simulink model "regcontrol_1ph"  (R2018b)
settings: Solver=VariableStepDiscrete  StartTime=0.0  StopTime=20.0  RelTol=1e-3
values from neighbouring files (symbols this model uses):
  BandWidth = Simulink.Parameter    [start.m]
  BaseVoltage = Simulink.Parameter    [start.m]
  CogenEnabled = false    [regcontrol_emulator.m]    (also in start.m = Simulink.Parameter)
  ElementTerminal = 0    [start.m]
  FPTphase = Simulink.Parameter(FPTphases.DEFAULT)    [regcontrol_emulator.m]    (also in start.m = 1)
  InCogenMode = false    [regcontrol_emulator.m]
  InReverseMode = false    [regcontrol_emulator.m]
  IsReversible = Simulink.Parameter    [start.m]
  LDC_Z = Simulink.Parameter    [start.m]
  MaxTap = 1.10    (= 1.1)    [Transformer.m]
  MinTap = 0.90    (= 0.9)    [Transformer.m]
  PTratio = Simulink.Parameter    [start.m]
  R = 0    [start.m]
  RevBand = Simulink.Parameter    [start.m]
  RevVreg = Simulink.Parameter    [start.m]
  TapLimitPerChange = Simulink.Parameter    [start.m]
  UsingRegulatedBus = Simulink.Parameter    [start.m]
  Vlimit = Simulink.Parameter    [start.m]
  Vreg = Simulink.Parameter    [start.m]
  X = 0    [start.m]
undefined symbols (not defined in the file or in its folder): Armed, ControlledTransformerConnection, ControlledTransformerCurrents, ControlledTransformerPowers, ControlledTransformerVoltages, CTRating, DeltaDirection, Handle, IsInverseTime, LastQueue, LookingForward, m, n, NumConductors, NumPhases, PresentTap, RevBackHandle, RevDelay, ReversePending, RevHandle, revLDC_Z, RevPowerThreshold, revR, revX, TapDelay, TapIncrement, TapWinding, TimeDelay, TimeInSec, VTerminal
(part 1 of 2)
settings Model: Creator=Michael Girbino  LastModifiedBy=Michael Girbino
settings DebuggingCC: LibraryContextMissingDiagnostic=none  SFNoUnconditionalDefaultTransitionDiag=warning  SFOutputUsedAsStateInMooreChartDiag=warning
settings SFSimCC: SimUseLocalCustomCode=off
settings RTWCC: RTWUseLocalCustomCode=off

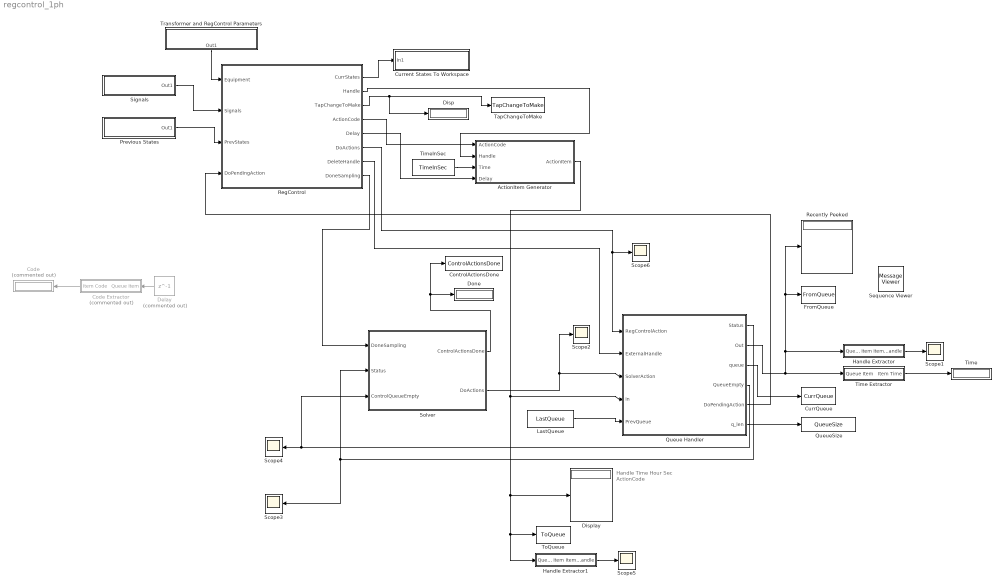
== system regcontrol_1ph ==
  note: Handle
      | Time
      | Hour
      | Sec
      | ActionCode
  ActionItem Generator : Subsystem
  Code : Display  Commented=on
  Code Extractor : Subsystem  Commented=on
  ControlActionsDone : ToWorkspace  VariableName=ControlActionsDone  SaveFormat=Timeseries  SampleTime=-1
  CurrQueue : ToWorkspace  VariableName=CurrQueue  SaveFormat=Structure With Time  SampleTime=1
  Current States To Workspace : Subsystem
  Delay : Delay  Commented=on  DelayLength=1  InitialCondition=0
  Disp : Display
  Display : Display
  Done : Display
  FromQueue : ToWorkspace  VariableName=FromQueue  SaveFormat=Structure With Time  SampleTime=1
  Handle Extractor : Subsystem
  Handle Extractor1 : Subsystem
  LastQueue : Constant  Value=LastQueue  VectorParams1D=off  OutDataTypeStr=double
  Previous States : Subsystem
  Queue Handler : Stateflow chart  TreatAsAtomicUnit=on
  QueueSize : ToWorkspace  VariableName=QueueSize  SaveFormat=Timeseries  SampleTime=-1
      settings: MaxDataPoints=1
  Recently Peeked : Display
  RegControl : Stateflow chart  TreatAsAtomicUnit=on
  Scope{1..6} (6 alike) : Scope
  Sequence Viewer : MessageViewer
  Signals : Subsystem
  Solver : Stateflow chart  TreatAsAtomicUnit=on
  TapChangeToMake : ToWorkspace  VariableName=TapChangeToMake  SaveFormat=Timeseries  SampleTime=-1
      settings: MaxDataPoints=1
  Time : Display
  Time Extractor : Subsystem
  TimeInSec : Constant  Value=TimeInSec  OutDataTypeStr=double
  ToQueue : ToWorkspace  VariableName=ToQueue  SaveFormat=Structure With Time  SampleTime=1
  Transformer and RegControl Parameters : Subsystem
  wires:
  Solver/2(DoActions) -> Scope2/1, Queue Handler/3(SolverAction)
  Queue Handler/1(Status) -> Scope3/1, Solver/2(Status)
  Queue Handler/3(queue) -> CurrQueue/1
  ActionItem Generator/1(ActionItem) -> ToQueue/1, Handle Extractor1/1(Queue Item), Display/1, Queue Handler/4(In)
  Solver/1(ControlActionsDone) -> ControlActionsDone/1, Done/1
  Queue Handler/4(QueueEmpty) -> Solver/3(ControlQueueEmpty), Scope4/1
  TimeInSec/1 -> ActionItem Generator/3(Time)
  LastQueue/1 -> Queue Handler/5(PrevQueue)
  Time Extractor/1(Item Time) -> Time/1
  RegControl/3(TapChangeToMake) -> Disp/1, TapChangeToMake/1
  Queue Handler/2(Out) -> Time Extractor/1(Queue Item), Handle Extractor/1(Queue Item), FromQueue/1, Recently Peeked/1
  Transformer and RegControl Parameters/1(Out1) -> RegControl/1(Equipment)
  RegControl/5(Delay) -> ActionItem Generator/4(Delay)
  Queue Handler/5(DoPendingAction) -> RegControl/4(DoPendingAction)
  RegControl/2(Handle) -> ActionItem Generator/2(Handle)
  RegControl/4(ActionCode) -> ActionItem Generator/1(ActionCode)
  RegControl/8(DoneSampling) -> Solver/1(DoneSampling)
  Signals/1(Out1) -> RegControl/2(Signals)
  Code Extractor/1(Item Code) -> Code/1
  Delay/1 -> Code Extractor/1(Queue Item)
  RegControl/7(DeleteHandle) -> Queue Handler/2(ExternalHandle)
  Previous States/1(Out1) -> RegControl/3(PrevStates)
  RegControl/1(CurrStates) -> Current States To Workspace/1(In1)
  Handle Extractor/1(Item Handle) -> Scope1/1
  Handle Extractor1/1(Item Handle) -> Scope5/1
  RegControl/6(DoActions) -> Scope6/1, Queue Handler/1(RegControlAction)
  Queue Handler/6(q_len) -> QueueSize/1

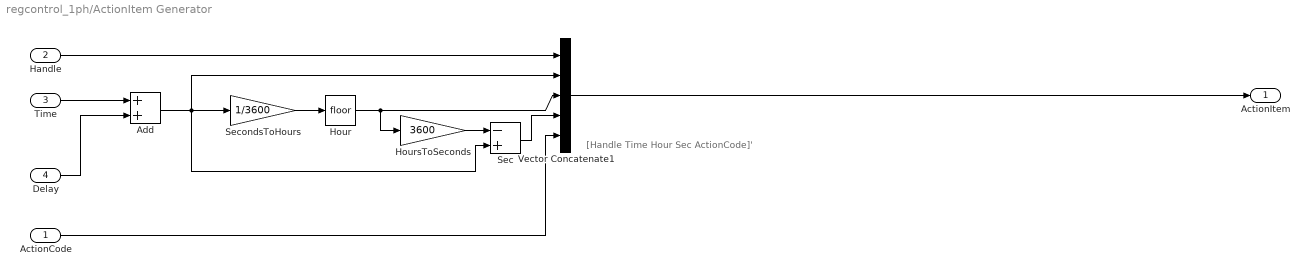
== system regcontrol_1ph/ActionItem Generator ==
  note: [Handle Time Hour Sec ActionCode]'
  ActionCode : Inport
  Handle : Inport  Port=2
  Time : Inport  Port=3
  Delay : Inport  Port=4
  Add : Sum
  Hour : Rounding
  HoursToSeconds : Gain  Gain=3600
  Sec : Sum  Inputs=-+
  SecondsToHours : Gain  Gain=1/3600
  Vector Concatenate1 : Concatenate  NumInputs=5
  ActionItem : Outport
  wires:
  Time/1 -> Add/1
  Hour/1 -> Vector Concatenate1/3, HoursToSeconds/1
  SecondsToHours/1 -> Hour/1
  Vector Concatenate1/1 -> ActionItem/1
  HoursToSeconds/1 -> Sec/1
  Handle/1 -> Vector Concatenate1/1
  Sec/1 -> Vector Concatenate1/4
  ActionCode/1 -> Vector Concatenate1/5
  Delay/1 -> Add/2
  Add/1 -> Sec/2, SecondsToHours/1, Vector Concatenate1/2

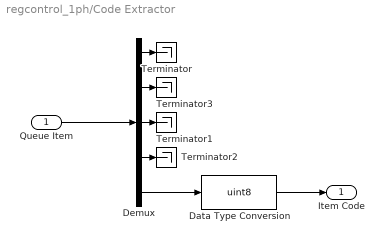
== system regcontrol_1ph/Code Extractor ==
  Queue Item : Inport
  Data Type Conversion : DataTypeConversion  OutDataTypeStr=uint8
  Demux : Demux  Outputs=5
  Terminator{,1..3} (4 alike) : Terminator
  Item Code : Outport
  wires:
  Demux/3 -> Terminator1/1
  Demux/4 -> Terminator2/1
  Demux/1 -> Terminator/1
  Queue Item/1 -> Demux/1
  Demux/5 -> Data Type Conversion/1
  Demux/2 -> Terminator3/1
  Data Type Conversion/1 -> Item Code/1

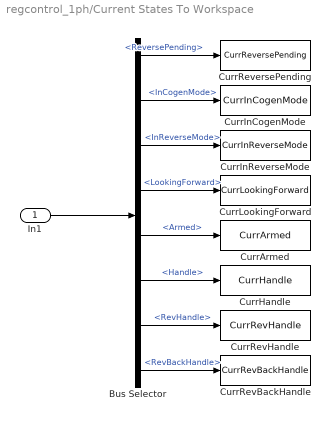
== system regcontrol_1ph/Current States To Workspace ==
  In1 : Inport
  Bus Selector : BusSelector  OutputSignals=ReversePending,InCogenMode,InReverseMode,LookingForward,Armed,Handle,RevHandle,RevBackHandle
  CurrArmed : ToWorkspace  VariableName=CurrArmed  SaveFormat=Timeseries  SampleTime=-1
      settings: MaxDataPoints=1
  CurrHandle : ToWorkspace  VariableName=CurrHandle  SaveFormat=Timeseries  SampleTime=-1
      settings: MaxDataPoints=1
  CurrInCogenMode : ToWorkspace  VariableName=CurrInCogenMode  SaveFormat=Timeseries  SampleTime=-1
      settings: MaxDataPoints=1
  CurrInReverseMode : ToWorkspace  VariableName=CurrInReverseMode  SaveFormat=Timeseries  SampleTime=-1
      settings: MaxDataPoints=1
  CurrLookingForward : ToWorkspace  VariableName=CurrLookingForward  SaveFormat=Timeseries  SampleTime=-1
      settings: MaxDataPoints=1
  CurrRevBackHandle : ToWorkspace  VariableName=CurrRevBackHandle  SaveFormat=Timeseries  SampleTime=-1
      settings: MaxDataPoints=1
  CurrRevHandle : ToWorkspace  VariableName=CurrRevHandle  SaveFormat=Timeseries  SampleTime=-1
      settings: MaxDataPoints=1
  CurrReversePending : ToWorkspace  VariableName=CurrReversePending  SaveFormat=Timeseries  SampleTime=-1
      settings: MaxDataPoints=1
  wires:
  In1/1 -> Bus Selector/1
  Bus Selector/1 -> CurrReversePending/1  "<ReversePending>"
  Bus Selector/2 -> CurrInCogenMode/1  "<InCogenMode>"
  Bus Selector/3 -> CurrInReverseMode/1  "<InReverseMode>"
  Bus Selector/4 -> CurrLookingForward/1  "<LookingForward>"
  Bus Selector/5 -> CurrArmed/1  "<Armed>"
  Bus Selector/6 -> CurrHandle/1  "<Handle>"
  Bus Selector/7 -> CurrRevHandle/1  "<RevHandle>"
  Bus Selector/8 -> CurrRevBackHandle/1  "<RevBackHandle>"

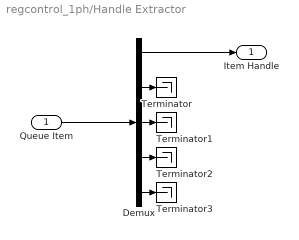
== system regcontrol_1ph/Handle Extractor ==
  Queue Item : Inport
  Demux : Demux  Outputs=5
  Terminator{,1..3} (4 alike) : Terminator
  Item Handle : Outport
  wires:
  Queue Item/1 -> Demux/1
  Demux/4 -> Terminator2/1
  Demux/3 -> Terminator1/1
  Demux/5 -> Terminator3/1
  Demux/1 -> Item Handle/1
  Demux/2 -> Terminator/1

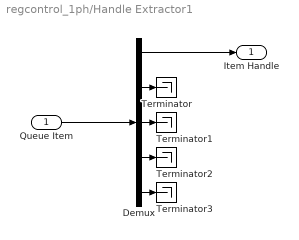
== system regcontrol_1ph/Handle Extractor1 ==
  Queue Item : Inport
  Demux : Demux  Outputs=5
  Terminator{,1..3} (4 alike) : Terminator
  Item Handle : Outport
  wires:
  Demux/2 -> Terminator/1
  Demux/1 -> Item Handle/1
  Demux/5 -> Terminator3/1
  Demux/3 -> Terminator1/1
  Demux/4 -> Terminator2/1
  Queue Item/1 -> Demux/1

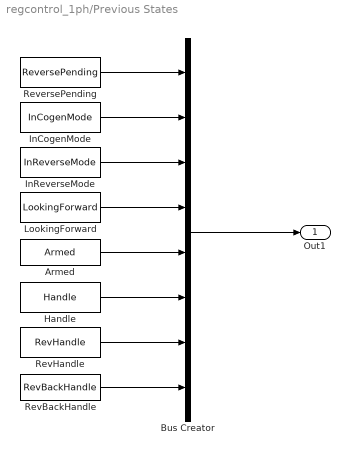
== system regcontrol_1ph/Previous States ==
  Armed : Constant  Value=Armed
  Bus Creator : BusCreator  Inputs=8  OutDataTypeStr=Bus: StatesBus
      settings: InheritFromInputs=off
  Handle : Constant  Value=Handle
  InCogenMode : Constant  Value=InCogenMode
  InReverseMode : Constant  Value=InReverseMode
  LookingForward : Constant  Value=LookingForward
  RevBackHandle : Constant  Value=RevBackHandle
  RevHandle : Constant  Value=RevHandle
  ReversePending : Constant  Value=ReversePending
  Out1 : Outport
  wires:
  Bus Creator/1 -> Out1/1
  ReversePending/1 -> Bus Creator/1
  InCogenMode/1 -> Bus Creator/2
  InReverseMode/1 -> Bus Creator/3
  LookingForward/1 -> Bus Creator/4
  Armed/1 -> Bus Creator/5
  Handle/1 -> Bus Creator/6
  RevHandle/1 -> Bus Creator/7
  RevBackHandle/1 -> Bus Creator/8

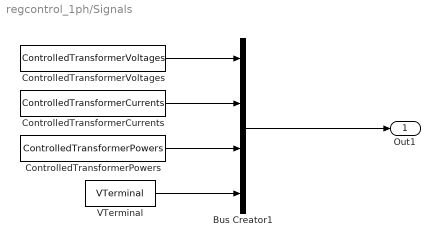
== system regcontrol_1ph/Signals ==
  Bus Creator1 : BusCreator  Inputs=4  OutDataTypeStr=Bus: SignalBus
      settings: InheritFromInputs=off
  ControlledTransformerCurrents : Constant  Value=ControlledTransformerCurrents
  ControlledTransformerPowers : Constant  Value=ControlledTransformerPowers
  ControlledTransformerVoltages : Constant  Value=ControlledTransformerVoltages
  VTerminal : Constant  Value=VTerminal
  Out1 : Outport
  wires:
  Bus Creator1/1 -> Out1/1
  ControlledTransformerPowers/1 -> Bus Creator1/3
  ControlledTransformerVoltages/1 -> Bus Creator1/1
  ControlledTransformerCurrents/1 -> Bus Creator1/2
  VTerminal/1 -> Bus Creator1/4

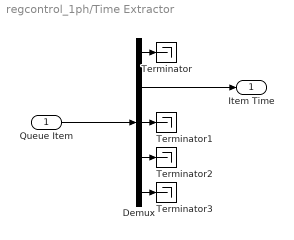
== system regcontrol_1ph/Time Extractor ==
  Queue Item : Inport
  Demux : Demux  Outputs=5
  Terminator{,1..3} (4 alike) : Terminator
  Item Time : Outport
  wires:
  Demux/5 -> Terminator3/1
  Demux/3 -> Terminator1/1
  Demux/4 -> Terminator2/1
  Demux/1 -> Terminator/1
  Demux/2 -> Item Time/1
  Queue Item/1 -> Demux/1

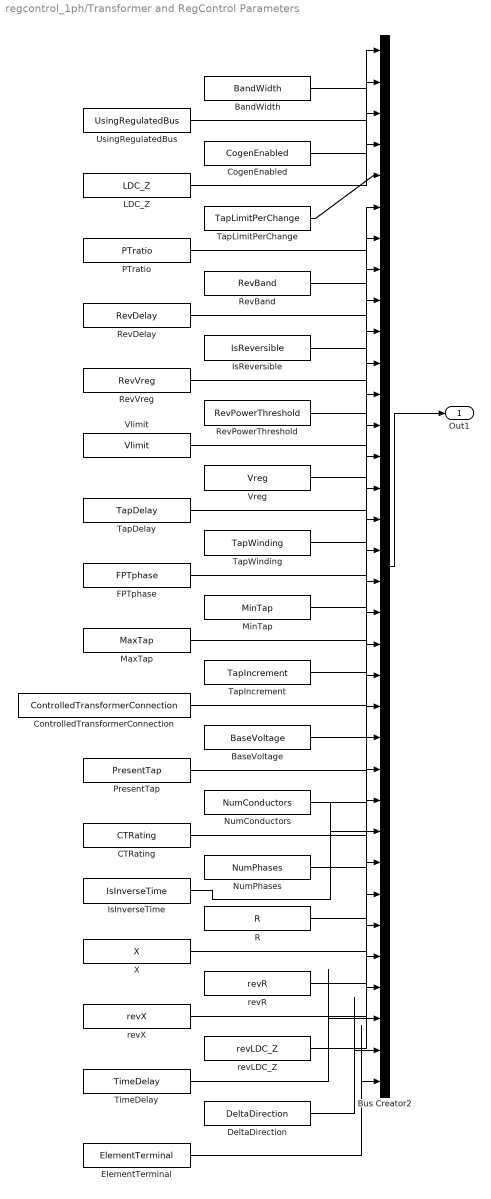
== system regcontrol_1ph/Transformer and RegControl Parameters ==
  BandWidth : Constant  Value=BandWidth
  BaseVoltage : Constant  Value=BaseVoltage
  Bus Creator2 : BusCreator  Inputs=34  OutDataTypeStr=Bus: EquipmentBus
      settings: InheritFromInputs=off
  CTRating : Constant  Value=CTRating
  CogenEnabled : Constant  Value=CogenEnabled
  ControlledTransformerConnection : Constant  Value=ControlledTransformerConnection
  DeltaDirection : Constant  Value=DeltaDirection
  ElementTerminal : Constant  Value=ElementTerminal
  FPTphase : Constant  Value=FPTphase
  IsInverseTime : Constant  Value=IsInverseTime
  IsReversible : Constant  Value=IsReversible
  LDC_Z : Constant  Value=LDC_Z
  MaxTap : Constant  Value=MaxTap
  MinTap : Constant  Value=MinTap
  NumConductors : Constant  Value=NumConductors
  NumPhases : Constant  Value=NumPhases
  PTratio : Constant  Value=PTratio
  PresentTap : Constant  Value=PresentTap
  R : Constant  Value=R
  RevBand : Constant  Value=RevBand
  RevDelay : Constant  Value=RevDelay
  RevPowerThreshold : Constant  Value=RevPowerThreshold
  RevVreg : Constant  Value=RevVreg
  TapDelay : Constant  Value=TapDelay
  TapIncrement : Constant  Value=TapIncrement
  TapLimitPerChange : Constant  Value=TapLimitPerChange
  TapWinding : Constant  Value=TapWinding
  TimeDelay : Constant  Value=TimeDelay
  UsingRegulatedBus : Constant  Value=UsingRegulatedBus
  Vlimit : Constant  Value=Vlimit
  Vreg : Constant  Value=Vreg
  X : Constant  Value=X
  revLDC_Z : Constant  Value=revLDC_Z
  revR : Constant  Value=revR
  revX : Constant  Value=revX
  Out1 : Outport
  wires:
  UsingRegulatedBus/1 -> Bus Creator2/2
  BandWidth/1 -> Bus Creator2/1
  TapWinding/1 -> Bus Creator2/15
  TapDelay/1 -> Bus Creator2/14
  Vreg/1 -> Bus Creator2/13
  Vlimit/1 -> Bus Creator2/12
  RevPowerThreshold/1 -> Bus Creator2/11
  RevVreg/1 -> Bus Creator2/10
  IsReversible/1 -> Bus Creator2/9
  RevDelay/1 -> Bus Creator2/8
  RevBand/1 -> Bus Creator2/7
  PTratio/1 -> Bus Creator2/6
  TapLimitPerChange/1 -> Bus Creator2/5
  LDC_Z/1 -> Bus Creator2/4
  CogenEnabled/1 -> Bus Creator2/3
  Bus Creator2/1 -> Out1/1
  FPTphase/1 -> Bus Creator2/16
  MinTap/1 -> Bus Creator2/17
  MaxTap/1 -> Bus Creator2/18
  TapIncrement/1 -> Bus Creator2/19
  ControlledTransformerConnection/1 -> Bus Creator2/20
  BaseVoltage/1 -> Bus Creator2/21
  PresentTap/1 -> Bus Creator2/22
  NumConductors/1 -> Bus Creator2/23
  CTRating/1 -> Bus Creator2/24
  NumPhases/1 -> Bus Creator2/25
  revLDC_Z/1 -> Bus Creator2/31
  revX/1 -> Bus Creator2/30
  revR/1 -> Bus Creator2/29
  X/1 -> Bus Creator2/28
  R/1 -> Bus Creator2/27
  IsInverseTime/1 -> Bus Creator2/26
  TimeDelay/1 -> Bus Creator2/32
  DeltaDirection/1 -> Bus Creator2/33
  ElementTerminal/1 -> Bus Creator2/34

== stateflow chart regcontrol_1ph/RegControl ==
  settings: enableNonTerminalStates=1
  state MakingTapChange [parallel] [commented out]
    state StaticTapChange [commented out]
      (default) -> (junction 165) [commented out] : {TapChangeToMake = AtLeastOneTap(LocalPendingTapChange, TapIncrement);
          | % reset to no change = change - 1 program will determin if another is needed:
          | LocalPendingTapChange = 0;
          | UpdateArmed(false);}
    state Finished [commented out]
      en: EXIT_TAPCHANGE = true;
    (default) -> (junction 132) [commented out]
    (junction 132) -> (junction 133) [commented out] : % Check to make sure control has not reset:
        | [LocalPendingTapChange == 0]
    (junction 132) -> (junction 163) [commented out]
    (junction 133) -> (junction 135) [commented out] : {UpdateArmed(false);}
    (junction 163) -> StaticTapChange [commented out] : [ControlMode == ControlModes.STATIC]
    (junction 163) -> MakingTapChange.Finished [commented out]
    StaticTapChange -> MakingTapChange.Finished [commented out]
    (junction 135) -> MakingTapChange.Finished [commented out]
  state Sampling [parallel]
    settings: executionOrder=1
    state DetermineReversePendingLookingForward
      state CorrectFalseReversePending
        en:
        if FwdPower < (-1*RevPowerThreshold)
        ReversePending = true;
        DeleteHandle = ...
        Push(ActionCodes.ACTION_REVERSE, ...
        RevDelay);
        RevHandle = DeleteHandle;
        end
      state CorrectTrueReversePending
        en:
        if FwdPower >= (-1*RevPowerThreshold)
        DeleteHandle = RevHandle;
        ReversePending = false;
        DoActions.data = QueueActions.DELETE;
        send(DoActions);
        RevHandle = 0;
        end
      state Finished
        en: GET_VOLTAGE = true;
      (default) -> (junction 599) : {FwdPower = ...
          | -1*real( sum( ControlledTransformerPower((TerminalOffset+1):...
          | (TerminalOffset+NumConductors)) ) );}
          | % Should we reverse?
      (junction 599) -> Sampling.DetermineReversePendingLookingForward.CorrectFalseReversePending [order 1] : [~ReversePending]
      (junction 599) -> (junction 646) [order 2]
      Sampling.DetermineReversePendingLookingForward.CorrectFalseReversePending -> (junction 646)
      (junction 646) -> (junction 594)
      (junction 594) -> Sampling.DetermineReversePendingLookingForward.CorrectTrueReversePending [order 1] : [ReversePending]
      (junction 594) -> (junction 654) [order 2]
      Sampling.DetermineReversePendingLookingForward.CorrectTrueReversePending -> (junction 654)
      (junction 654) -> Sampling.DetermineReversePendingLookingForward.Finished
    state DetermineReversePendingLookingReverseOrCogen
      state CorrectFalseReversePending
        en:
        if FwdPower > RevPowerThreshold
        ReversePending = true;
        % push Reverse Back action to switch back:
        DeleteHandle = ...
        Push(ActionCodes.ACTION_REVERSE, ...
        RevDelay);
        RevBackHandle = DeleteHandle;
        end
      state CorrectTrueReversePending
        en:
        if FwdPower <= RevPowerThreshold
        DeleteHandle = RevBackHandle;
        ReversePending = false;
        % delete Reverse Back action:
        DoActions.data = QueueActions.DELETE;
        send(DoActions);
        RevBackHandle = 0;
        end
      state Finished
        en: REV_NEUTRAL = true;
      (default) -> (junction 620) : {FwdPower = ...
          | -1*real( sum( ControlledTransformerPower((TerminalOffset+1):...
          | (TerminalOffset+NumConductors)) ) );}
          | % If reversed, check if power is back in forward direction
      (junction 620) -> Sampling.DetermineReversePendingLookingReverseOrCogen.CorrectFalseReversePending [order 1] : [~ReversePending]
      (junction 620) -> (junction 621) [order 2]
      Sampling.DetermineReversePendingLookingReverseOrCogen.CorrectFalseReversePending -> (junction 621)
      (junction 621) -> (junction 624)
      (junction 624) -> Sampling.DetermineReversePendingLookingReverseOrCogen.CorrectTrueReversePending [order 1] : [ReversePending]
      (junction 624) -> (junction 650) [order 2]
      Sampling.DetermineReversePendingLookingReverseOrCogen.CorrectTrueReversePending -> (junction 650)
      (junction 650) -> Sampling.DetermineReversePendingLookingReverseOrCogen.Finished
    state ReverseNeutralCase
      state Finished
        en:
        GET_VOLTAGE = true;
      state ReverseNeutralTapChange
        en:
        PendingTapChange = ...
        round( (1.0 - double(TapWinding)) / TapIncrement ) * TapIncrement;
        if PendingTapChange ~= 0.0 && ~Armed
        Push(ActionCodes.ACTION_TAPCHANGE, TapDelay);
        Armed = true;
        end
      state Exiting
        en: EXIT = true;
      (default) -> (junction 592)
      (junction 592) -> (junction 637) [order 1] : % tap change not specified as needed:
          | [~Armed]
      (junction 592) -> Sampling.ReverseNeutralCase.Finished [order 2]
      (junction 637) -> (junction 614) : {PendingTapChange = 0.0;}
      (junction 614) -> (junction 638) [order 1] : [abs(PresentTap - 1.0) < EPSILON]
      (junction 614) -> Exiting [order 2]
      (junction 638) -> ReverseNeutralTapChange
      ReverseNeutralTapChange -> (junction 649)
      (junction 649) -> Exiting
    state GetVoltage
      en:
      if UsingRegulatedBus
      GetRegulatedBusVoltage; % stores voltages in VBuffer
      else
      VBuffer = ControlledTransformerWindingVoltages((TerminalOffset+1):(TerminalOffset+NumPhases));
      end
      Vcontrol = GetControlVoltage; % operates on VBuffer
    state DetermineVlocalbus
      state Finished
        en: GET_VOLTAGEWLDC = true;
      (default) -> (junction 689)
      (junction 689) -> (junction 691) [order 1] : % Voltage limit for bus connected to regulated winding; default = 0.0 (inactive)
          | [VlimitActive]
      (junction 689) -> Sampling.DetermineVlocalbus.Finished [order 2] : {Vlocalbus = 0.0;}
      (junction 691) -> (junction 683)
      (junction 683) -> (junction 692) [order 1] : % when controlled transformer is different from LDC PTransformer
          | [UsingRegulatedBus]
      (junction 683) -> (junction 696) [order 2] : % controlled transformer is
          | % the LDC PTransformer
          | {Vlocalbus = abs(Vcontrol);}
      (junction 692) -> (junction 714) : {%ControlledTransformer.GetWindingVoltages(ElementTerminal, VBuffer);
          | Vlocalbus = abs( VBuffer(1) / PTRatio );}
      (junction 714) -> (junction 696)
      (junction 696) -> (junction 675)
      (junction 675) -> Sampling.DetermineVlocalbus.Finished
    state GetVoltageWithLDC
      state RX_LDCmode
        en:
        if InReverseMode || InCogenMode
        VLDC = complex(revR, revX) * ...
        complex( real(ILDC), imag(ILDC) );
        else
        VLDC = complex(R, X) * ...
        complex( real(ILDC), imag(ILDC) );
        end
      state Z_LDCmode
        en:
        if InReverseMode || InCogenMode
        Vcontrol = abs(Vcontrol) - abs(ILDC) * revLDC_Z;
        else
        Vcontrol = abs(Vcontrol) - abs(ILDC) * LDC_Z;
        end
      state Finished
        en: GET_TEST_VALUES = true;
      (default) -> (junction 771) : {% Convert current to control current by CTRating:
          | ILDC = ControlledTransformerCurrents(TerminalOffset + ControlledPhase) / CTRating;}
      (junction 771) -> RX_LDCmode [order 1] : % Standard R, X LDC
          | [LDC_Z == 0.0]
      (junction 771) -> Z_LDCmode [order 2] : % Beckwith LDC_Z control mode
      RX_LDCmode -> (junction 872)
      Z_LDCmode -> Sampling.GetVoltageWithLDC.Finished
      (junction 872) -> Sampling.GetVoltageWithLDC.Finished
    state GetTestValues
      en:
      Vactual = abs(Vcontrol);
      if InReverseMode
      Vactual = Vactual / PresentTap;
      VregTest = RevVreg;
      BandTest = RevBandwidth;
      else
      VregTest = Vreg;
      BandTest = Bandwidth;
      end
    state DetermineTapChangeIsNeeded
      en:
      if abs(VregTest - Vactual) > BandTest/2.0
      TapChangeIsNeeded = true;
      else
      TapChangeIsNeeded = false;
      end
    state MakeTapChange
      state GetVboostFromVlimit
        en:
        if Vlocalbus > Vlimit
        Vboost = Vlimit - Vlocalbus;
        end
      state TapChangeUp
        en:
        if PresentTap < MaxTap
        Push(ActionCodes.ACTION_TAPCHANGE, ...
        ComputeTimeDelay(Vactual));
        Armed = true;
        end
      state TapChangeDown
        en:
        if PresentTap > MinTap
        Push(ActionCodes.ACTION_TAPCHANGE, ...
        ComputeTimeDelay(Vactual));
        Armed = true;
        end
      state Finished
        en: FINISHED = true;
      (default) -> (junction 720) : % compute tapchange:
          | {Vboost = VregTest - Vactual;}
      (junction 720) -> (junction 766) [order 1] : [VlimitActive]
      (junction 720) -> (junction 723) [order 2]
      (junction 766) -> GetVboostFromVlimit
      GetVboostFromVlimit -> (junction 724)
      (junction 724) -> (junction 723)
      (junction 723) -> (junction 728) : {% PU winding boost needed:
          | BoostNeeded = Vboost * PTRatio / BaseVoltage;
          | Increment = TapIncrement;
          | % quantize to an increment:
          | PendingTapChange = ...
          | round(BoostNeeded/Increment)*Increment;
          | }
      (junction 728) -> (junction 731) : % send initial tap change message to ControlQueue, add delay time to solution control queue:
      (junction 731) -> (junction 817) [order 1] : % only changes 1 tap at a time:
          | [PendingTapChange ~= 0.0 && ~Armed]
      (junction 731) -> Sampling.MakeTapChange.Finished [order 2]
      (junction 817) -> (junction 810) : % see of any tap change is possible in desired direction (not saturated):
      (junction 810) -> TapChangeUp [order 1] : % going up:
          | [PendingTapChange > 0.0]
      (junction 810) -> TapChangeDown [order 2]
      TapChangeUp -> (junction 819)
      TapChangeDown -> (junction 820)
      (junction 820) -> Sampling.MakeTapChange.Finished
      (junction 819) -> (junction 820)
    state Finished
      en:
      WriteStatesToOutput;
      send(DoneSampling);
    (default) -> (junction 822) : {AssignEquipmentToLocals;
        | AssignSignalsToLocals;
        | AssignStatesToLocals;}
    (junction 822) -> (junction 815) [order 1] : [TapLimitPerChange ~= 0]
    (junction 815) -> (junction 826)
    (junction 822) -> (junction 807) [order 2]
    (junction 826) -> (junction 823) [order 1] : [~UsingRegulatedBus]
    (junction 826) -> (junction 818) [order 2]
    (junction 823) -> (junction 787)
    (junction 787) -> (junction 832) [order 1] : [IsReversible || CogenEnabled]
    (junction 787) -> (junction 792) [order 2]
    (junction 832) -> (junction 828)
    (junction 828) -> DetermineReversePendingLookingForward [order 1] : [LookingForward && ~InCogenMode]
    (junction 828) -> DetermineReversePendingLookingReverseOrCogen [order 2]
    DetermineReversePendingLookingForward -> (junction 825) : [GET_VOLTAGE]
    DetermineReversePendingLookingReverseOrCogen -> (junction 844) : [REV_NEUTRAL]
    (junction 844) -> ReverseNeutralCase [order 1] : % mode for which tap change may be executed,
        | % but no reversal made:
        | [ReverseNeutral]
    (junction 844) -> (junction 806) [order 2]
    ReverseNeutralCase -> (junction 806) [order 2] : [GET_VOLTAGE]
    (junction 806) -> (junction 808)
    ReverseNeutralCase -> (junction 829) [order 1] : [EXIT]
    (junction 792) -> (junction 818)
    (junction 808) -> (junction 792)
    (junction 825) -> (junction 808)
    (junction 818) -> GetVoltage
    (junction 829) -> (junction 807)
    (junction 807) -> (junction 816)
    GetVoltage -> DetermineVlocalbus
    DetermineVlocalbus -> (junction 845) : [GET_VOLTAGEWLDC]
    (junction 845) -> GetVoltageWithLDC [order 1] : % line drop compensation, but not using regulated bus
        | [~UsingRegulatedBus && LDCActive]
    (junction 845) -> (junction 809) [order 2]
    GetVoltageWithLDC -> (junction 839) : [GET_TEST_VALUES]
    (junction 839) -> (junction 809)
    (junction 809) -> GetTestValues
    GetTestValues -> DetermineTapChangeIsNeeded
    DetermineTapChangeIsNeeded -> (junction 788)
    (junction 788) -> MakeTapChange [order 1] : [TapChangeIsNeeded]
    (junction 788) -> (junction 813) [order 2]
    MakeTapChange -> (junction 837) : [FINISHED]
    (junction 837) -> (junction 813)
    (junction 813) -> Sampling.Finished
    (junction 816) -> Sampling.Finished : {PendingTapChange = 0;}
  state Execution [parallel]
    settings: executionOrder=2
    state Asleep
    state ParseAction
      en: Code = DoPendingAction.data;
      discard(DoPendingAction);
      length(DoPendingAction);
    state MakingTapChange
      en:
      if PendingTapChange ~= 0
      TapChangeToMake = AtLeastOneTap(PendingTapChange);
      PendingTapChange = 0;
      Armed = false;
      end
    state Reversing
      state FlipCogen
        en:
        if InCogenMode
        InCogenMode = false;
        else
        InCogenMode = true;
        end
      state FlipReverse
        en:
        if InReverseMode
        InReverseMode = false;
        else
        InReverseMode = true;
        end
      state Finished
        en:
        ReversePending = false;
        EXIT_REVERSE = true;
      (default) -> (junction 229)
      (junction 229) -> (junction 230) [order 1] : [ReversePending]
      (junction 229) -> Execution.Reversing.Finished [order 2]
      (junction 230) -> (junction 242)
      (junction 242) -> (junction 238) [order 1] : [CogenEnabled]
      (junction 242) -> FlipReverse [order 2]
      (junction 238) -> FlipCogen : % Cogen mode takes precedence if present
      FlipReverse -> (junction 240)
      FlipCogen -> (junction 245)
      (junction 240) -> Execution.Reversing.Finished
      (junction 245) -> (junction 240)
    state Finished
      en: WriteStatesToOutput;
    (default) -> Asleep
    Asleep -> ParseAction : DoPendingAction
    ParseAction -> (junction 115)
    (junction 115) -> Execution.MakingTapChange [order 1] : [Code == ActionCodes.ACTION_TAPCHANGE]
    (junction 115) -> (junction 119) [order 2]
    Execution.MakingTapChange -> (junction 122)
    (junction 119) -> Reversing [order 1] : [Code == ActionCodes.ACTION_REVERSE]
    (junction 119) -> (junction 123) [order 2]
    Reversing -> (junction 122) : [EXIT_REVERSE]
    (junction 122) -> (junction 124)
    (junction 124) -> (junction 123)
    (junction 123) -> Execution.Finished
  state ChangeToMake = AtLeastOneTap(ProposedChange) [function]
    note: Called in STATIC mode
        | Changes 70% of the way but at least one tap, subject to maximum allowable tap change
    (default) -> (junction 283) : {NumTaps = floor(0.7 * abs(ProposedChange)/TapIncrement);}
    (junction 283) -> (junction 284) [order 1] : [NumTaps == 0]
    (junction 283) -> (junction 285) [order 2]
    (junction 284) -> (junction 286) : {NumTaps = 1.0;} % At least 1 tap
    (junction 286) -> (junction 285)
    (junction 285) -> (junction 293)
    (junction 293) -> (junction 290) [order 1] : [NumTaps > TapLimitPerChange]
    (junction 293) -> (junction 294) [order 2]
    (junction 290) -> (junction 295) : {NumTaps = double(TapLimitPerChange);} % Bound by maximum
    (junction 295) -> (junction 294)
    (junction 294) -> (junction 302) : {LastChange = NumTaps;}
    (junction 302) -> (junction 303) [order 1] : % Check sign on change:
        | [ProposedChange > 0]
    (junction 302) -> (junction 304) [order 2] : {ChangeToMake = ...
        | -1*double(NumTaps)*TapIncrement;
        | LastChange = -1*NumTaps;}
    (junction 303) -> (junction 305) : {ChangeToMake =...
        |  double(NumTaps)*TapIncrement;}
    (junction 305) -> (junction 304)
    (junction 304) -> (junction 306)
  state Result = GetControlVoltage [function]
    note: GetControlVoltage
        | Called when voltage is sampled from the same transformer whose taps are controlled.
        | Returns the voltage which will be used to decide tap changes. Also changes the ControlledPhase if it is different from FPTphase.
    note: FPTphase is max phase.
        |
        | VControl is taken from the phase with the greatest voltage.
        |
        | ControlledPhase becomes that phase.
    note: FPTphase is min phase.
        |
        | VControl is taken from the phase with the least voltage.
        |
        | ControlledPhase becomes that phase.
    (default) -> (junction 496)
    (junction 496) -> (junction 486) [order 1] : [FPTphase == uint8(FPTphases.MAXPHASE)]
        | % controlled phase is that with greatest |V|
    (junction 496) -> (junction 517) [order 2]
    (junction 486) -> (junction 523) : {ControlledPhase = 1;
        | % abs is equivalent to Cabs:
        | V = abs( VBuffer(ControlledPhase) );}
        | % Iteration through remaining phases:
    (junction 510) -> (junction 489) [order 1] : [ii <= NumPhases]
    (junction 489) -> (junction 485)
    (junction 523) -> (junction 510) : {ii = uint8(2);}
    (junction 485) -> (junction 515) [order 1] : [abs( VBuffer(ControlledPhase)) > V]
        | % if it's GREATER, make it the new V
    (junction 485) -> (junction 522) [order 2]
    (junction 515) -> (junction 516) : {V = abs( VBuffer(ii) );
        | ControlledPhase = ii;}
    (junction 487) -> (junction 510) : {ii = ii+1;}
    (junction 510) -> (junction 534) [order 2] : {Result = VBuffer(ControlledPhase) / PTRatio;
        | % Complex divided by real
        | }
    (junction 516) -> (junction 522)
    (junction 522) -> (junction 487)
    (junction 534) -> (junction 527)
    (junction 527) -> (junction 519)
    (junction 517) -> (junction 533) [order 1] : [FPTphase == uint8(FPTphases.MINPHASE)]
        | % controlled phase is that with least |V|
    (junction 533) -> (junction 535) : {ControlledPhase = 1;
        | % abs is equivalent to Cabs:
        | V = abs( VBuffer(ControlledPhase) );}
        | % Iteration through remaining phases:
    (junction 517) -> (junction 1027) [order 2] : % Default case: use specified phase,
        | % as long as it's feasible
    (junction 513) -> (junction 537) [order 1] : [ii <= NumPhases]
    (junction 537) -> (junction 488)
    (junction 535) -> (junction 513) : {ii = uint8(2);}
    (junction 1027) -> (junction 1028) [order 1] : [FPTphase > NumPhases]
    (junction 488) -> (junction 504) [order 1] : [abs( VBuffer(ControlledPhase)) < V]
        | % if it's LESS, make it the new V
    (junction 1027) -> (junction 1029) [order 2] : {FPTphase = max(FPTphase, 1);}
    (junction 1028) -> (junction 1030) : {FPTphase = 1;}
    (junction 488) -> (junction 514) [order 2]
    (junction 504) -> (junction 507) : {V = abs( VBuffer(ii) );
        | ControlledPhase = ii;}
    (junction 518) -> (junction 513) : {ii = ii+1;}
    (junction 513) -> (junction 536) [order 2] : {Result = VBuffer(ControlledPhase) / PTRatio;
        | % Complex divided by real
        | }
    (junction 507) -> (junction 514)
    (junction 514) -> (junction 518)
    (junction 1030) -> (junction 1029)
    (junction 1029) -> (junction 497) : {Result = VBuffer(FPTphase) / PTRatio;
        | ControlledPhase = FPTphase;}
    (junction 536) -> (junction 519)
    (junction 519) -> (junction 502)
    (junction 502) -> (junction 497)
    (junction 497) -> (junction 498)
  state Result = ComputeTimeDelay(Vavg) [function]
    (default) -> (junction 477)
    (junction 477) -> (junction 481) [order 1] : [IsInverseTime]
    (junction 477) -> (junction 482) [order 2] : % determines which regulator control will act first,
        | % default is 15s
        | {Result = TimeDelay;}
    (junction 481) -> (junction 483) : % TimeDelay is adjusted inversely proportional to
        | % the amount that voltage is outside the band,
        | % down to 10 percent of specified time delay
        | % (Further out of band = band - 1> less time delay)
        | {Result = TimeDelay / min(10.0, 2.0*abs(Vreg - Vavg)/Bandwidth);}
    (junction 483) -> (junction 482)
    (junction 482) -> (junction 474)
  state AssignEquipmentToLocals [function]
    (default) -> (junction 550) : {
        | BandWidth = Equipment.BandWidth;
        | UsingRegulatedBus = Equipment.UsingRegulatedBus;
        | CogenEnabled = Equipment.CogenEnabled;
        | LDC_Z = Equipment.LDC_Z;
        | TapLimitPerChange = Equipment.TapLimitPerChange;
        | PTRatio = Equipment.PTratio;
        | RevBand = Equipment.RevBand;
        | RevDelay = Equipment.RevDelay;
        | IsReversible = Equipment.IsReversible;
        | RevVreg = Equipment.RevVreg;
        | RevPowerThreshold = Equipment.RevPowerThreshold;
        | Vlimit = Equipment.Vlimit;
        | Vreg = Equipment.Vreg;
        | TapDelay = Equipment.TapDelay;
        | TapWinding = Equipment.TapWinding;
        | FPTphase = Equipment.FPTphase;
        |
        | MinTap = Equipment.MinTap;
        | MaxTap = Equipment.MaxTap;
        | TapIncrement = Equipment.TapIncrement;
        | ControlledTransformerConnection = Equipment.ControlledTransformerConnection;
        | BaseVoltage = Equipment.BaseVoltage;
        | NumConductors = Equipment.NumConductors;
        | NumPhases = Equipment.NumPhases;
        | CTRating = Equipment.CTRating;
        | IsInverseTime = Equipment.IsInverseTime;
        |
        | R = Equipment.R;
        | X = Equipment.X;
        | revR = Equipment.revR;
        | revX = Equipment.revX;
        | revLDC_Z = Equipment.revLDC_Z;
        | TimeDelay = Equipment.TimeDelay;
        |
        | % From Script:
        | TapWinding = Equipment.TapWinding;
        | TapIncrement = Equipment.TapIncrement;
        | TapDelay = Equipment.TapDelay;
        | CogenEnabled = Equipment.CogenEnabled;
        | PresentTap = Equipment.PresentTap;
        | TapLimitPerChange = Equipment.TapLimitPerChange;
        | ElementTerminal = Equipment.ElementTerminal;
        | DeltaDirection = Equipment.DeltaDirection;
        | }
    (junction 550) -> (junction 548) [order 1] : [R~=0 || X~=0 || LDC_Z ~=0]
    (junction 550) -> (junction 555) [order 2] : {LDCActive = false;}
    (junction 548) -> (junction 552) : {LDCActive = true;}
    (junction 552) -> (junction 555)
    (junction 555) -> (junction 547)
  state h = Push(CodeVal, DelayVal) [function]
    (default) -> (junction 462) : {ActionCode = double(CodeVal);
        | Delay = DelayVal;
        | DoActions.data = QueueActions.PUSH;
        | send(DoActions);
        | h = uint8(Handle);
        | Handle = Handle + double(1);
        | }
  state AssignSignalsToLocals [function]
    (default) -> (junction 940) : {ControlledTransformerWindingVoltages = Signals.ControlledTransformerVoltages;
        | ControlledTransformerPower = Signals.ControlledTransformerPowers;
        | ControlledTransformerCurrents = Signals.ControlledTransformerCurrents;
        | VTerminal = Signals.VTerminal;
        |
        | TerminalOffset = NumConductors*(ElementTerminal - 1);
        | VBuffer = zeros(NumPhases, 1);}
  state AssignStatesToLocals [function]
    (default) -> (junction 943) : {ReversePending = PrevStates.ReversePending;
        | InCogenMode = PrevStates.InCogenMode;
        | InReverseMode = PrevStates.InReverseMode;
        | LookingForward = PrevStates.LookingForward;
        | Armed = PrevStates.Armed;
        | Handle = double(PrevStates.Handle);
        | RevHandle = PrevStates.RevHandle;
        | RevBackHandle = PrevStates.RevBackHandle;
        | }
  state GetRegulatedBusVoltage [function]
    (junction 989) -> (junction 998) [order 1] : [ii <= NumPhases]
    (default) -> (junction 989) : {ii = uint8(1);}
    (junction 998) -> (junction 1002)
    (junction 1002) -> (junction 991) [order 1] : [ControlledTransformerConnection == Connections.DELTA]
    (junction 1002) -> (junction 1015) [order 2]
    (junction 991) -> (junction 992) : {rotIdx = RotatePhases(ii, NumPhases, DeltaDirection);
        | VBuffer(ii) = VTerminal(TerminalOffset+ii) - ...
        | VTerminal(TerminalOffset+rotIdx);}
    (junction 1015) -> (junction 1007) [order 1] : [ControlledTransformerConnection == ...
        | Connections.WYE]
    (junction 1015) -> (junction 1017) [order 2]
    (junction 1007) -> (junction 990) : {VBuffer(ii) = VTerminal(TerminalOffset+ii);}
    (junction 997) -> (junction 989) : {ii = ii+1;}
    (junction 989) -> (junction 1005) [order 2]
    (junction 990) -> (junction 1017)
    (junction 992) -> (junction 990)
    (junction 1017) -> (junction 997)
  state WriteStatesToOutput [function]
    (default) -> (junction 947) : {CurrStates.ReversePending = ReversePending;
        | CurrStates.InCogenMode = InCogenMode;
        | CurrStates.InReverseMode = InReverseMode;
        | CurrStates.LookingForward = LookingForward;
        | CurrStates.Armed = Armed;
        | CurrStates.Handle = uint8(Handle);
        | CurrStates.RevHandle = RevHandle;
        | CurrStates.RevBackHandle = RevBackHandle;
        | }
  data: ProposedChange function_input; ChangeToMake function_output; NumTaps local double; Result function_output; Vavg function_input; Result function_output; CodeVal function_input; DelayVal function_input; h function_output; idx function_input; newIdx function_output; NPhases function_input; DeltaDir function_input; CurrStates output Bus: StatesBus; Equipment input Bus: EquipmentBus; Signals input Bus: SignalBus; PrevStates input Bus: StatesBus; Handle output double =0; EXIT_REVERSE local boolean =false; InReverseMode local boolean =false; ReversePending local boolean; InCogenMode local boolean =false; DoPendingAction input double; TapWinding local uint8; TapIncrement local double; TapDelay local double; CogenEnabled local boolean =false; TapChangeToMake output double; PendingTapChange local double =double(0); TapLimitPerChange local uint8 =uint8(16); ActionCode output double; Delay output double =0; DoActions output Enum: QueueActions; DeleteHandle output uint8 size=[1] =uint8(0); DoneSampling output boolean =true; Armed local boolean =false; PresentTap local double; Vactual local double =0; Vcontrol local double =complex(0); FPTphase local uint8 size=[1]; VBuffer local double size=[3 1]; NumPhases local uint8 size=[1]; ControlledPhase local uint8 size=[1] =uint8(1); PTRatio local double =60; IsInverseTime local boolean; TimeDelay local double; Vreg local double =120; Bandwidth local double =3; revR local double =0; RevVreg local double =120; revX local double =0; ControlledTransformerConnection local uint8 size=[1]; ControlledTransformerCurrents local double; ControlledTransformerPower local double; ControlledTransformerWindingVoltages local double size=[4 1]; CTRating local double; MaxTap local double; MinTap local double; Vlimit local double =0; RevDelay local double; revLDC_Z local double =0; RevPowerThreshold local double; RevBandwidth local double =3; ElementTerminal local uint8 size=[1] =uint8(1); LDCActive local boolean =false; VlimitActive local boolean =false; Increment local double =0; IsReversible local boolean =false; LookingForward local boolean =false; ReverseNeutral local boolean =false; NumConductors local uint8 size=[1]; BaseVoltage local double; UsingRegulatedBus local boolean =false; VLDC local double =complex(0); FINISHED local boolean =false; VregTest local double =0; BandTest local double =0; EXIT local boolean =false; ILDC local double =complex(0); Vboost local double =0; FwdPower local double =0; GET_TEST_VALUES local boolean =false; GET_VOLTAGE local boolean =false; GET_VOLTAGEWLDC local boolean =false; Vlocalbus local double =0; BoostNeeded local double =0; RevBackHandle local uint8 size=[1] =uint8(0); REV_NEUTRAL local boolean =false; TapChangeIsNeeded local boolean =false; LDC_Z local double =0; R local double =0; X local double =0; EPSILON local double =1.0e-12; RevHandle local uint8 size=[1] =uint8(0); LastChange local double; DeltaDirection local uint8; VTerminal local double size=[4 1]; TerminalOffset local uint8 =uint8(0); Code local double size=[1 1]
  function newIdx = RotatePhases(idx, NPhases, DeltaDir):
    | function newIdx = RotatePhases(idx, NPhases, DeltaDir)
    |     dd = int8(1);
    |     
    |     switch(DeltaDir)
    |         case DeltaDirs.FORWARD
    |             dd = int8(1);
    |         case DeltaDirs.REVERSE
    |             dd = int8(-1);
    |     end
    | 
    |     newIdx = uint8( int8(idx) + dd );
    | 
    |     % make sure RotatedPhase is within limits:
    |     if NPhases > 2
    |         % Assumes 2 phase delta is open delta
    |         if newIdx > NPhases
    |             newIdx = uint8(1);
    |         elseif newIdx < 1
    |             newIdx = NPhases;
    |         end
    |     elseif newIdx < 1
    |         newIdx = uint8(3); % For 2-phase delta, next phase will be 3rd phase
    |     end
    | end

== stateflow chart regcontrol_1ph/Solver ==
  state ControlFlow [parallel]
    settings: executionOrder=1
    state Asleep
    note: Static
        | - dummy QueueTime
        | - DoNearestActions
    state SolverFinished
    (default) -> ControlFlow.Asleep
    ControlFlow.Asleep -> (junction 54) : DoneSampling
    (junction 54) -> (junction 55) [order 1] : [LocalControlQueueEmpty]
        | % execute nearest set of control actions, but leave time where it is
    (junction 54) -> (junction 56) [order 2] : {DoActions.data = QueueActions.DO_NEAREST_ACTIONS;
        | send(DoActions);
        | % ignores time advancement
        | }
    (junction 55) -> (junction 57) : {ControlActionsDone = true;}
    (junction 57) -> (junction 56)
    (junction 56) -> SolverFinished
  state CheckIfEmpty [parallel]
    settings: executionOrder=2
    state Asleep
    state QueueEmptyCase
      en: LocalControlQueueEmpty = true;
    (default) -> CheckIfEmpty.Asleep
    CheckIfEmpty.Asleep -> QueueEmptyCase : ControlQueueEmpty
  data: DoneSampling input boolean; ControlActionsDone output boolean; DoActions output Enum: QueueActions; Status input Enum: Statuses; LocalControlQueueEmpty local boolean =false; ControlQueueEmpty input boolean
